simulink model "demoOtterUSVHeadingControl"  (R2021a)
settings: Solver=ode4  StartTime=0.0  StopTime=50  FixedStep=0.05  RelTol=1e-3
libraries: mssSimulink x3, simulink x1
settings Model: Creator=thor  LastModifiedBy=thor

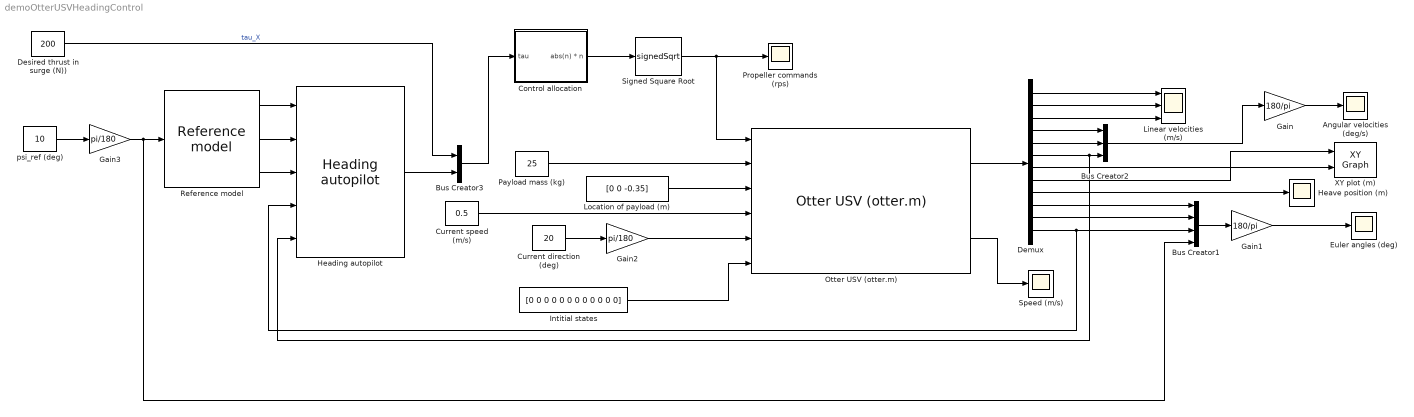
== system demoOtterUSVHeadingControl ==
  Angular velocities (deg/s) : Scope
  Bus Creator1 : BusCreator  Inputs=4
  Bus Creator2 : BusCreator  Inputs=3
  Bus Creator3 : BusCreator  Inputs=2
  Control allocation : Subsystem
  Current direction (deg) : Constant  Value=20
  Current speed (m/s) : Constant  Value=0.5
  Demux : Demux  Outputs=12
  Desired thrust in surge (N)) : Constant  Value=200
  Euler angles (deg) : Scope
  Gain : Gain  Gain=180/pi
  Gain1 : Gain  Gain=180/pi
  Gain2 : Gain  Gain=pi/180
  Gain3 : Gain  Gain=pi/180
  "Heading autopilot " : mssSimulink/Control/Autopilots/Heading autopilot  T_nomoto=5  K_nomoto=1  Kp=300  Td=1  Ti=10
  Heave position (m) : Scope
  Intitial states : Constant  Value=[0 0 0 0 0 0 0 0 0 0 0 0]
  Linear velocities (m/s) : Scope  NumInputPorts=3
  Location of payload (m) : Constant  Value=[0 0 -0.35]
  "Otter USV (otter.m) " : mssSimulink/Marine craft models/Otter USV (otter.m)  SystemSampleTime=-1  VariantActivationTime=update diagram  Latency=0  AutoFrameSizeCalculation=off
  Payload mass (kg) : Constant  Value=25
  Propeller commands (rps) : Scope
  Reference model : mssSimulink/Guidance/Reference model  v_max=10  zeta_d=1.0  w_d=1
  Signed Square Root : Sqrt  Operator=signedSqrt  SaturateOnIntegerOverflow=on
  Speed (m/s) : Scope
  XY plot (m) : simulink/Sinks/XY Graph  xmin=-20  xmax=20  ymin=-20  ymax=20  st=-1
  psi_ref (deg) : Constant  Value=10
  wires:
  Demux/8 -> XY plot (m)/1
  Demux/7 -> XY plot (m)/2
  Demux/1 -> Linear velocities (m/s)/1
  Demux/2 -> Linear velocities (m/s)/2
  Demux/3 -> Linear velocities (m/s)/3
  Demux/10 -> Bus Creator1/1
  Demux/11 -> Bus Creator1/2
  Demux/4 -> Bus Creator2/1
  Demux/5 -> Bus Creator2/2
  Bus Creator2/1 -> Gain/1
  Demux/9 -> Heave position (m)/1
  Payload mass (kg)/1 -> "Otter USV (otter.m) "/2
  Location of payload (m)/1 -> "Otter USV (otter.m) "/3
  Current speed (m/s)/1 -> "Otter USV (otter.m) "/4
  Current direction (deg)/1 -> Gain2/1
  Intitial states/1 -> "Otter USV (otter.m) "/6
  "Otter USV (otter.m) "/1 -> Demux/1
  "Otter USV (otter.m) "/2 -> Speed (m/s)/1
  Gain/1 -> Angular velocities (deg/s)/1
  Gain1/1 -> Euler angles (deg)/1
  Gain2/1 -> "Otter USV (otter.m) "/5
  "Heading autopilot "/1 -> Bus Creator3/2
  Demux/12 -> "Heading autopilot "/4, Bus Creator1/3
  Demux/6 -> "Heading autopilot "/5, Bus Creator2/3
  Desired thrust in surge (N))/1 -> Bus Creator3/1  "tau_X"
  Reference model/1 -> "Heading autopilot "/1
  Reference model/2 -> "Heading autopilot "/2
  Reference model/3 -> "Heading autopilot "/3
  psi_ref (deg)/1 -> Gain3/1
  Gain3/1 -> Bus Creator1/4, Reference model/1
  Bus Creator1/1 -> Gain1/1
  Signed Square Root/1 -> "Otter USV (otter.m) "/1, Propeller commands (rps)/1
  Bus Creator3/1 -> Control allocation/1(tau)
  Control allocation/1(abs(n) * n) -> Signed Square Root/1

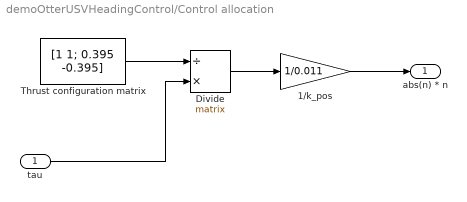
== system demoOtterUSVHeadingControl/Control allocation ==
  tau : Inport
  1/k_pos : Gain  Gain=1/0.011
  Divide : Product  Inputs=/*  Multiplication=Matrix(*)
  Thrust configuration matrix : Constant  Value=[1 1; 0.395 -0.395]
  abs(n) * n : Outport
  wires:
  tau/1 -> Divide/2
  Divide/1 -> 1/k_pos/1
  1/k_pos/1 -> abs(n) * n/1
  Thrust configuration matrix/1 -> Divide/1
